simulink model "working_final_model"  (R2023b)
settings: Solver=VariableStepAuto  StartTime=0.0  StopTime=inf  RelTol=1e-3
libraries: spsSeriesRLCLoadLib x7, spsIdealSwitchLib x6, spsRMSLib x3, eePowerMeasurement x2, spsVoltageMeasurementLib x2, spsCurrentMeasurementLib x1, spsSeriesRLCBranchLib x1, spsACVoltageSourceLib x1, spsVariableInductorLib x1, spsVariableResistorLib x1, sps_lib x1
settings Model: Creator=ASUS  LastModifiedBy=ASUS

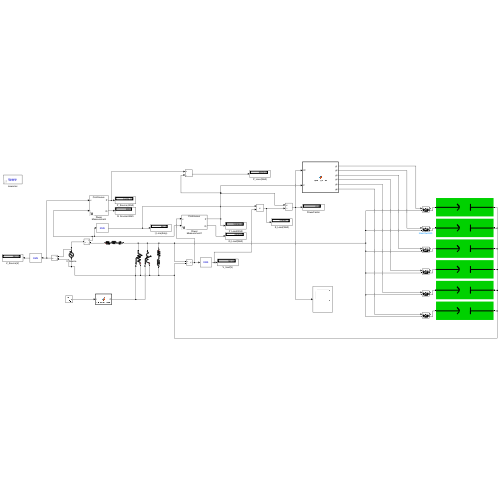
[thumbnail: Simulink's stored preview of the top-level diagram]
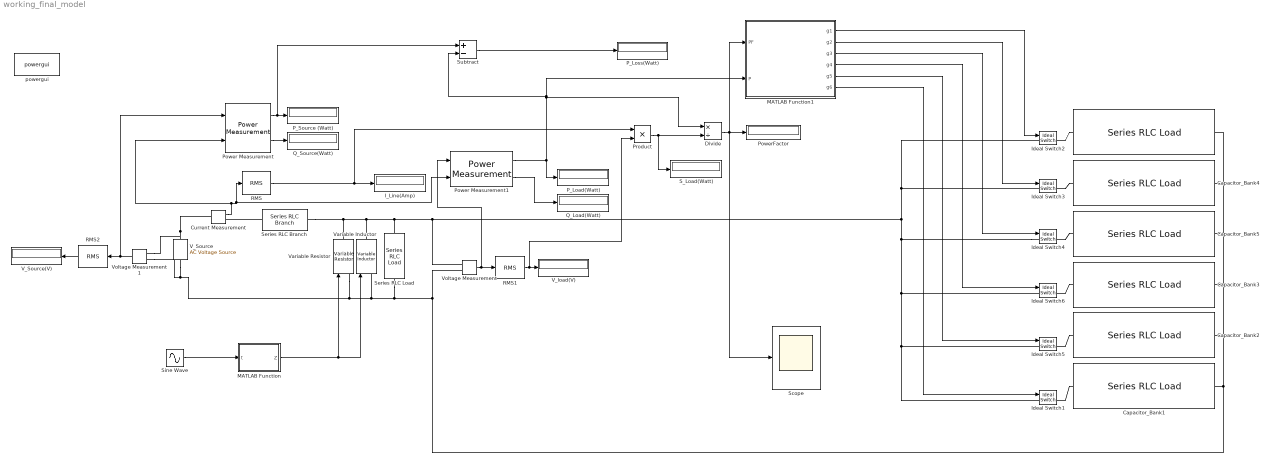
== system working_final_model ==
  " " : spsSeriesRLCLoadLib/Series RLC Load  LConnTagsString=a  RConnTagsString=__new0  NominalVoltage=120  NominalFrequency=60  ActivePower=0  InductivePower=0  CapacitivePower=500  Setx0=off  InitialVoltage=0  SetiL0=off  InitialCurrent=0  Measurements=None  LoadType=constant Z
  Capacitor_Bank{1..5} (5 alike) : spsSeriesRLCLoadLib/Series RLC Load  LConnTagsString=a  RConnTagsString=__new0  NominalVoltage=120  NominalFrequency=60  ActivePower=0  InductivePower=0  CapacitivePower=500  Setx0=off  InitialVoltage=0  SetiL0=off  InitialCurrent=0  Measurements=None  LoadType=constant Z
  Current Measurement : spsCurrentMeasurementLib/Current Measurement  PhasorSimulation=off  OutputType=Complex  PSBequivalent=0
  Divide : Product  Inputs=*/
  I_Line(Amp) : Display
  Ideal Switch{1..6} (6 alike) : spsIdealSwitchLib/Ideal Switch  Ron=0.0001  Lon=0  IC=0  Rs=1e5  Cs=inf  Measurements=on
  MATLAB Function : MATLAB Function  TreatAsAtomicUnit=on
  MATLAB Function1 : MATLAB Function  TreatAsAtomicUnit=on
  P_Load(Watt) : Display
      settings: Format=bank
  P_Loss(Watt) : Display
      settings: Format=bank
  P_Source (Watt) : Display
      settings: Format=bank
  Power Measurement : eePowerMeasurement/Power Measurement  LabelModeActiveChoice=Continuous  F=60  K=[1]  Ts=0
  Power Measurement1 : eePowerMeasurement/Power Measurement  LabelModeActiveChoice=Continuous  F=60  K=[1]  Ts=0
  PowerFactor : Display
      settings: Format=bank
  Product : Product
  Q_Load(Watt) : Display
      settings: Format=bank
  Q_Source(Watt) : Display
  RMS : spsRMSLib/RMS  TrueRMS=on  Freq=60  RMSInit=120  Ts=0
  RMS1 : spsRMSLib/RMS  TrueRMS=on  Freq=60  RMSInit=120  Ts=0
  RMS2 : spsRMSLib/RMS  TrueRMS=on  Freq=60  RMSInit=120  Ts=0
  S_Load(Watt) : Display
      settings: Format=bank
  Scope : Scope
  Series RLC Branch : spsSeriesRLCBranchLib/Series RLC Branch  LConnTagsString=__new0  RConnTagsString=__new0  BranchType=RLC  Resistance=1  Inductance=0  SetiL0=off  InitialCurrent=0  Capacitance=0  Setx0=off  InitialVoltage=0  Measurements=None
  Series RLC Load : spsSeriesRLCLoadLib/Series RLC Load  LConnTagsString=a  RConnTagsString=__new0  NominalVoltage=120  NominalFrequency=60  ActivePower=3000  InductivePower=2250  CapacitivePower=0  Setx0=off  InitialVoltage=0  SetiL0=off  InitialCurrent=0  Measurements=None  LoadType=constant Z
  Sine Wave : Sin  SampleTime=0
  Subtract : Sum  Inputs=+-
  V_Source : spsACVoltageSourceLib/AC Voltage Source  Amplitude=240*sqrt(2)  Phase=0  Frequency=60  SampleTime=0  Measurements=None  BusType=swing  Pref=10e3  Qref=0  Qmin=-inf  Qmax=+inf
  V_Source(V) : Display
      settings: Format=bank
  V_load(V) : Display
      settings: Format=bank
  Variable Inductor : spsVariableInductorLib/Variable Inductor  methode=Backward Euler  Labsmin=1e-6  Initialize=off  iL0=0  L0=1e-3  Vl0=-35.7214
      settings: LibrarySourceBlock=sps_lib/Passives/Variable Inductor
  Variable Resistor : spsVariableResistorLib/Variable Resistor  Rabsmin=1e-3
      settings: LibrarySourceBlock=sps_lib/Passives/Variable Resistor
  Voltage Measurement : spsVoltageMeasurementLib/Voltage Measurement  PhasorSimulation=off  OutputType=Complex  PSBequivalent=0
  Voltage Measurement1 : spsVoltageMeasurementLib/Voltage Measurement  PhasorSimulation=off  OutputType=Complex  PSBequivalent=0
  powergui : sps_lib/powergui  Priority=1  SimulationMode=Discrete  SampleTime=50e-6  frequency=60  Iterations=50  frequencyindice=60  Pbase=100e6  ErrMax=1e-4  UnitsV=kV  UnitsW=MW  buscounter=0  FunctionMessages=off  echomessages=off  EnableUseOfTLC=off  CurrentSourceSwitches=off  DisableSnubberDevices=off  DisableRonSwitches=off  DisableVfSwitches=off  DisplayEquations=off  AutomaticDiscreteSolvers=off  SolverType=Tustin/Backward Euler (TBE)  Interpol=off  ExternalGateDelay=off  methode=off  Ts=100  x0status=blocks  SPID=on  SwTol=0  HookPort=off  NonlinearTolerance=1e-4  nMaxIteration=100  ContinueOnMaxIteration=off  RestoreLinks=warning  ResistiveCurrentMeasurement=off  Frange=[0:2:500]  Ylog=off  Xlog=on  ShowGrid=off  save=off  variable=ZData  structure=0  ZoomFFT=off  StartTime=0.0  cycles=1  DisplayStyle=1  fundamental=60  FreqAxis=off  MaxFrequency=1000  frequencyindicesteady=1  RmsSteady=1  display=off
  wires:
  MATLAB Function1/2(g2) -> Ideal Switch3/1
  Divide/1 -> Scope/1, MATLAB Function1/1(PF), PowerFactor/1
  Product/1 -> S_Load(Watt)/1, Divide/2
  RMS/1 -> Product/1, I_Line(Amp)/1
  MATLAB Function/1(Z) -> Variable Inductor/1, Variable Resistor/1
  Subtract/1 -> P_Loss(Watt)/1
  Power Measurement1/2 -> Q_Load(Watt)/1
  Power Measurement/2 -> Q_Source(Watt)/1
  Power Measurement1/1 -> MATLAB Function1/2(P), Subtract/2, Divide/1, P_Load(Watt)/1
  Sine Wave/1 -> MATLAB Function/1(t)
  RMS1/1 -> Product/2, V_load(V)/1
  Current Measurement/1 -> RMS/1, Power Measurement1/2, Power Measurement/2
  MATLAB Function1/6(g6) -> Ideal Switch1/1
  Voltage Measurement1/1 -> Power Measurement/1, RMS2/1
  Power Measurement/1 -> Subtract/1, P_Source (Watt)/1
  RMS2/1 -> V_Source(V)/1
  MATLAB Function1/4(g4) -> Ideal Switch6/1
  Voltage Measurement/1 -> Power Measurement1/1, RMS1/1
  MATLAB Function1/1(g1) -> Ideal Switch2/1
  MATLAB Function1/3(g3) -> Ideal Switch4/1
  MATLAB Function1/5(g5) -> Ideal Switch5/1
  connections:
  Capacitor_Bank5/LConn1 -- Variable Resistor/LConn1 -- V_Source/LConn1 -- Voltage Measurement1/LConn2 -- Variable Inductor/LConn1 -- Series RLC Load/RConn1 -- Voltage Measurement/LConn2 -- Capacitor_Bank1/LConn1 -- Capacitor_Bank2/LConn1 -- Capacitor_Bank3/LConn1 -- " "/LConn1 -- Capacitor_Bank4/LConn1
  Ideal Switch4/LConn1 -- Ideal Switch5/LConn1 -- Ideal Switch1/LConn1 -- Ideal Switch6/LConn1 -- Series RLC Branch/RConn1 -- Variable Resistor/RConn1 -- Variable Inductor/RConn1 -- Series RLC Load/LConn1 -- Voltage Measurement/LConn1 -- Ideal Switch3/LConn1 -- Ideal Switch2/LConn1
  Voltage Measurement1/LConn1 -- V_Source/RConn1 -- Current Measurement/LConn1
  Ideal Switch6/RConn1 -- Capacitor_Bank3/RConn1
  Ideal Switch1/RConn1 -- Capacitor_Bank1/RConn1
  Ideal Switch4/RConn1 -- Capacitor_Bank5/RConn1
  Ideal Switch5/RConn1 -- Capacitor_Bank2/RConn1
  Ideal Switch2/RConn1 -- " "/RConn1
  Ideal Switch3/RConn1 -- Capacitor_Bank4/RConn1
  Series RLC Branch/LConn1 -- Current Measurement/RConn1

== matlab function working_final_model/MATLAB Function1 ==
  data: g1 output; PF input; P input; g2 output; g3 output; g4 output; g5 output; g6 output
function [g1, g2, g3, g4, g5, g6] = gate_control(PF, P)
%#codegen
% Control 6 capacitor banks based on power factor and real power

    cap_VAR = 500;       % Each capacitor provides 500 VAR
    total_caps = 6;
    PF_target = 0.99;

    theta_b = acos(PF);
    theta_t = acos(PF_target);
    Q_required = P * (tan(theta_b) - tan(theta_t));  % in VAR

    % Number of capacitors needed
    num_on = min(ceil(Q_required / cap_VAR), total_caps);

    % Initialize all gates to 0
    gates = zeros(1, 6);
    gates(1:num_on) = 1;  % Turn ON required no. of banks

    % Assign outputs
    [g1, g2, g3, g4, g5, g6] = deal(gates(1), gates(2), gates(3), gates(4), gates(5), gates(6));
end

== matlab function working_final_model/MATLAB Function ==
  data: t input; Z output
function Z = variable_load(t)
    Z = 10 + 5*sin(2*pi*0.5*t); % Load varies smoothly
end
